simulink model "rlMultipleFirstOrderLagSystem"  (R2020a)
settings: Solver=FixedStepAuto  StartTime=0.0  StopTime=10.0  FixedStep=0.01  RelTol=1e-3
model workspace (MAT data in the model file):
  K1 = 1
  K2 = 0.9
  Sig = Simulink.Signal
  Sig.DataType = 'auto'
  Sig.Dimensions = -1
  Sig.DimensionsMode = 'auto'
  Sig.Complexity = 'auto'
  Sig.SampleTime = -1
  Sig.SamplingMode = 'auto'
  T1 = 0.05
  T2 = 0.1
  x0 = 0
libraries: cstblocks x1, rllib x1
settings Model: Creator=Student  LastModifiedBy=Student

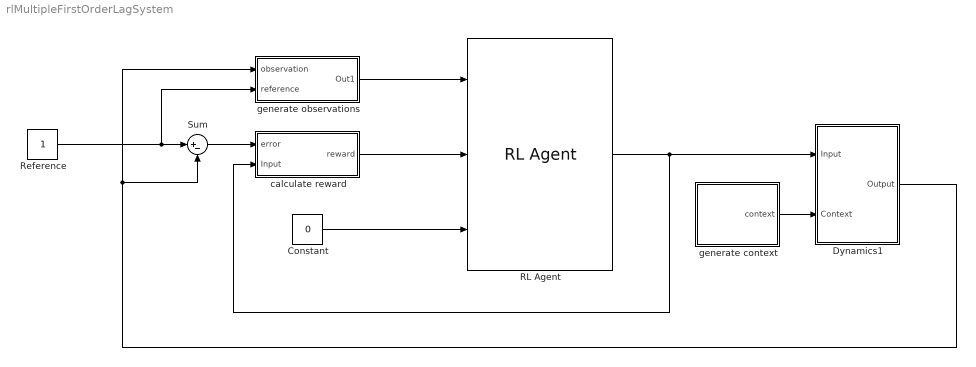
== system rlMultipleFirstOrderLagSystem ==
  Constant : Constant  Value=0
  Dynamics1 : Subsystem
  RL Agent : rllib/RL Agent  Agent=agent  ProvideReward=on  ProvideIsDone=on  ProvideCumRwd=off  TreatAsDirectFeedthrough=on  CollectLoggedSignals=on  CollectModelStates=on
  Reference : Constant
  Sum : Sum  Inputs=|+-
  calculate reward : Subsystem
  generate context : Subsystem
  generate observations : Subsystem
  wires:
  generate context/1(context) -> Dynamics1/2(Context)
  Reference/1 -> generate observations/2(reference), Sum/1
  Sum/1 -> calculate reward/1(error)
  Dynamics1/1("Output ") -> generate observations/1(observation), Sum/2
  calculate reward/1(reward) -> RL Agent/2
  RL Agent/1 -> Dynamics1/1("Input "), calculate reward/2("Input ")
  Constant/1 -> RL Agent/3
  generate observations/1(Out1) -> RL Agent/1

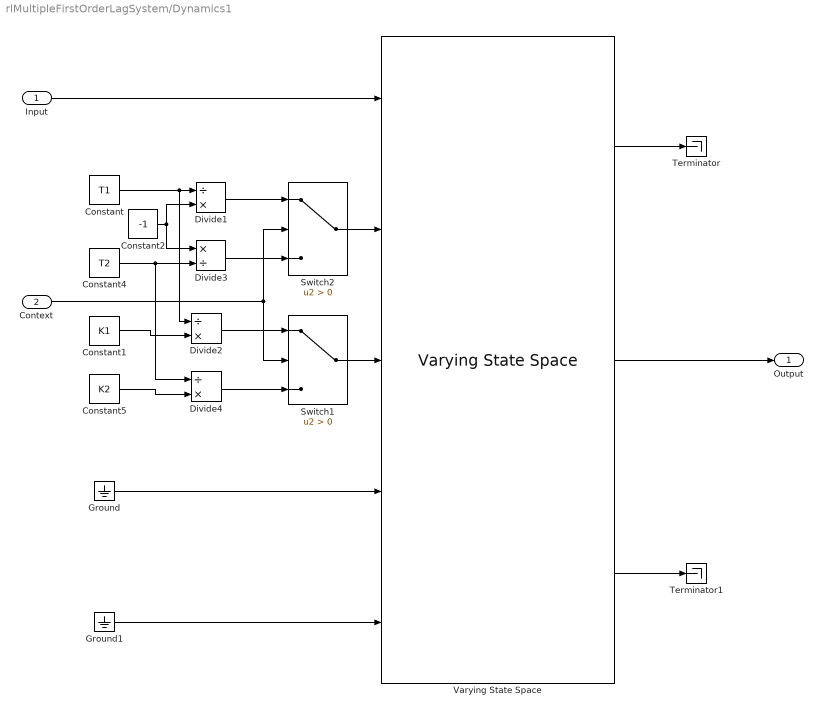
== system rlMultipleFirstOrderLagSystem/Dynamics1 ==
  "Input " : Inport
  Context : Inport  Port=2
  Constant : Constant  Value=T1
  Constant1 : Constant  Value=K1
  Constant2 : Constant  Value=-1
  Constant4 : Constant  Value=T2
  Constant5 : Constant  Value=K2
  Divide1 : Product  Inputs=/*
  Divide2 : Product  Inputs=/*
  Divide3 : Product  Inputs=*/
  Divide4 : Product  Inputs=/*
  Ground : Ground
  Ground1 : Ground
  Switch1 : Switch  Criteria=u2 > Threshold
  Switch2 : Switch  Criteria=u2 > Threshold
  Terminator : Terminator
  Terminator1 : Terminator
  Varying State Space : cstblocks/Linear Parameter Varying/Varying State Space  x0=x0  xNames=''  OutputX=on  OutputDX=on
  "Output " : Outport
  wires:
  Switch1/1 -> Varying State Space/3
  Divide3/1 -> Switch2/3
  Varying State Space/2 -> "Output "/1
  Constant/1 -> Divide2/1, Divide1/1
  Context/1 -> Switch1/2, Switch2/2
  Switch2/1 -> Varying State Space/2
  Divide1/1 -> Switch2/1
  "Input "/1 -> Varying State Space/1
  Constant2/1 -> Divide3/1, Divide1/2
  Constant4/1 -> Divide4/1, Divide3/2
  Varying State Space/1 -> Terminator/1
  Varying State Space/3 -> Terminator1/1
  Ground/1 -> Varying State Space/4
  Ground1/1 -> Varying State Space/5
  Constant1/1 -> Divide2/2
  Divide2/1 -> Switch1/1
  Divide4/1 -> Switch1/3
  Constant5/1 -> Divide4/2

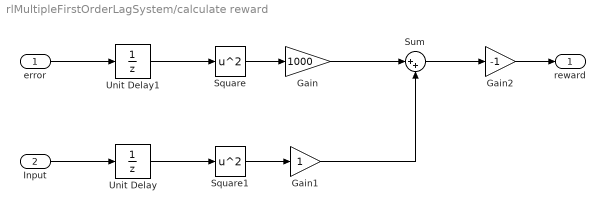
== system rlMultipleFirstOrderLagSystem/calculate reward ==
  error : Inport
  "Input " : Inport  Port=2
  Gain : Gain  Gain=1000
  Gain1 : Gain
  Gain2 : Gain  Gain=-1
  Square : Math  Operator=square  SaturateOnIntegerOverflow=on
  Square1 : Math  Operator=square  SaturateOnIntegerOverflow=on
  Sum : Sum  Inputs=|++
  Unit Delay : UnitDelay  SampleTime=-1  HasFrameUpgradeWarning=on
  Unit Delay1 : UnitDelay  InitialCondition=1  SampleTime=-1  HasFrameUpgradeWarning=on
  reward : Outport
  wires:
  Square/1 -> Gain/1
  Gain1/1 -> Sum/2
  Gain/1 -> Sum/1
  Sum/1 -> Gain2/1
  Gain2/1 -> reward/1
  "Input "/1 -> Unit Delay/1
  Unit Delay/1 -> Square1/1
  Square1/1 -> Gain1/1
  error/1 -> Unit Delay1/1
  Unit Delay1/1 -> Square/1

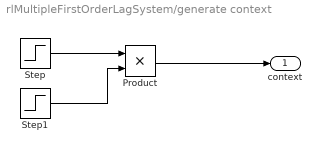
== system rlMultipleFirstOrderLagSystem/generate context ==
  Product : Product
  Step : Step  Time=5  SampleTime=0
  Step1 : Step  Time=10  Before=1  After=0  SampleTime=0
  context : Outport
  wires:
  Step/1 -> Product/1
  Step1/1 -> Product/2
  Product/1 -> context/1

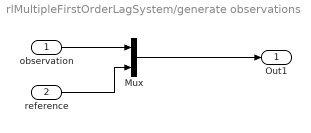
== system rlMultipleFirstOrderLagSystem/generate observations ==
  observation : Inport
  reference : Inport  Port=2
  Mux : Mux  Inputs=2
  Out1 : Outport
  wires:
  observation/1 -> Mux/1
  reference/1 -> Mux/2
  Mux/1 -> Out1/1
